simulink model "TP2_R3FMO_ctrl_2016"  (R2017b)
settings: Solver=ode23s  StartTime=0.0  StopTime=.15  RelTol=1e-3  EnableMultiTasking=on
values from neighbouring files (symbols this model uses):
  anchoPulso = 5    [TP2_R3FMO_ctrl_2016.m]    (also in TP2_R3FMO_ctrl_2016_p_2.m = 40; TP2_R3FMO_ctrl_2016_p_3.m = 40)
  t1 = fase1+theta    (= 0.00666666666667)    [TP2_R3FMO_ctrl_2016.m]    (also in TP2_R3FMO_ctrl_2016_p_2.m = 0.005; TP2_R3FMO_ctrl_2016_p_3.m = 0.005)
  t2 = fase2+theta    (= 0.0133333333333)    [TP2_R3FMO_ctrl_2016.m]    (also in TP2_R3FMO_ctrl_2016_p_2.m = 0.0116666666667; TP2_R3FMO_ctrl_2016_p_3.m = 0.0116666666667)
  t3 = fase3+theta    (= 0.02)    [TP2_R3FMO_ctrl_2016.m]    (also in TP2_R3FMO_ctrl_2016_p_2.m = 0.0183333333333; TP2_R3FMO_ctrl_2016_p_3.m = 0.0183333333333)
  tCorto = 0.075    [TP2_R3FMO_ctrl_2016.m]    (also in TP2_R3FMO_ctrl_2016_p_2.m = 0.028; TP2_R3FMO_ctrl_2016_p_3.m = 0.028)
libraries: powerlib x11, powerlib_meascontrol x2
settings Model: Creator=Moni  LastModifiedBy=Sebastián
settings DataIOCC: SaveFormat=Array  SaveState=on
settings OptimizationCC: LifeSpan=inf
settings DebuggingCC: SolverPrmCheckMsg=warning  SFUnexpectedBacktrackingDiag=warning  SFNoUnconditionalDefaultTransitionDiag=warning  SFExecutionAtInitializationDiag=none
settings HardwareCC: ProdBitPerPointer=32  ProdBitPerSizeT=32  ProdBitPerPtrDiffT=32  ProdLargestAtomicFloat=None  ProdIntDivRoundTo=Undefined  ProdEndianess=Unspecified  ProdWordSize=32  ProdHWDeviceType=32-bit Generic
settings ModelReferenceCC: PropagateSignalLabelsOutOfModel=off
settings CodeAppCC: StateflowObjectComments=on
settings GRTTargetCC: TargetLangStandard=C89/C90 (ANSI)  GeneratePreprocessorConditionals=Disable all
settings ConfigComp: CovMetricSettings=dw  CovHtmlReporting=on  CovSaveCumulativeToWorkspaceVar=on  CovSaveSingleToWorkspaceVar=on  CovExternalEMLEnable=off  CovSFcnEnable=off
settings SimscapeCC: SimscapeNormalizeSystem=off

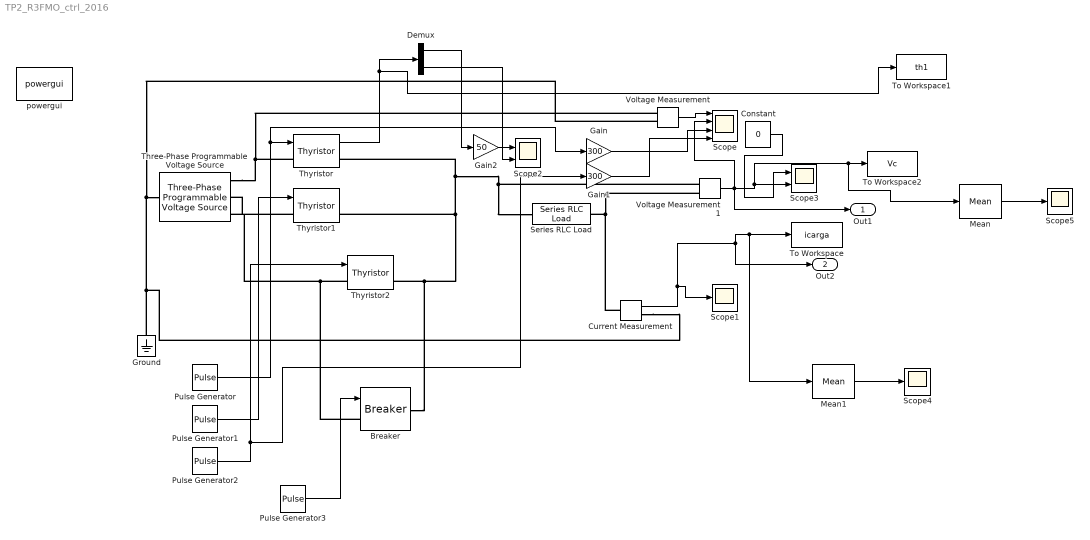
== system TP2_R3FMO_ctrl_2016 ==
  Breaker : powerlib/Elements/Breaker  InitialState=0  SwitchingTimes="[1/60  5/60]"  External=on  BreakerResistance=0.01  SnubberResistance=1e6  SnubberCapacitance=inf  Measurements=None  MoreParameters=on  NoBreakLoop=off
      settings: SourceProductName=Simscape Power Systems
  Constant : Constant  Value=0
  Current Measurement : powerlib/Measurements/Current Measurement  PhasorSimulation=off  OutputType=Complex  PSBequivalent=0
  Demux : Demux  Outputs=2
  Gain : Gain  Gain=300
  Gain1 : Gain  Gain=300
  Gain2 : Gain  Gain=50
  Ground : powerlib/Elements/Ground  LConnTagsString=a
  Mean : powerlib_meascontrol/Measurements/Mean  Freq=50  Vinit=0  Ts=0
  Mean1 : powerlib_meascontrol/Measurements/Mean  Freq=50  Vinit=0  Ts=0
  Pulse Generator : DiscretePulseGenerator  PulseType=Time based  Period=.02  PulseWidth=anchoPulso  PhaseDelay=t1
  Pulse Generator1 : DiscretePulseGenerator  PulseType=Time based  Period=.02  PulseWidth=anchoPulso  PhaseDelay=t2
  Pulse Generator2 : DiscretePulseGenerator  PulseType=Time based  Period=.02  PulseWidth=anchoPulso  PhaseDelay=t3
  Pulse Generator3 : DiscretePulseGenerator  PulseType=Time based  Period=10  PulseWidth=99  PhaseDelay=tCorto
  Scope : Scope  NumInputPorts=4
  Scope1 : Scope
  Scope2 : Scope  NumInputPorts=2
  Scope3 : Scope  NumInputPorts=2
  Scope4 : Scope
  Scope5 : Scope
  Series RLC Load : powerlib/Elements/Series RLC Load  LConnTagsString=a  RConnTagsString=__new0  NominalVoltage=220  NominalFrequency=50  ActivePower=100  InductivePower=Q  CapacitivePower=0  Setx0=off  InitialVoltage=0  SetiL0=off  InitialCurrent=0  Measurements=None  LoadType=constant Z
  Three-Phase Programmable Voltage Source : powerlib/Electrical Sources/Three-Phase Programmable Voltage Source  PositiveSequence="[380  0 50]"  VariationEntity=None  VariationType=Table of time-amplitude pairs  VariationTypeAlt=Step  VariationStep=0.5  VariationRate=10  VariationMagnitude=0.3  VariationFrequency=2  VariationTiming=[1 2]  VariationPhaseA=off  Amplitudes=[1 0.8 1.2 1.0]  TimeValues=[0 0.1 0.15 0.2]  HarmonicGeneration=off  HarmonicA=[3 0.2 -25 0]  HarmonicB=[2 0.15 35 2]  Timing="[0.05  3]"  BusType=swing  Pref=0  Qref=0  Qmin=-inf  Qmax=inf
  Thyristor : powerlib/Power Electronics/Thyristor  Ron=0.001  Lon=0  Vf=0.8  IC=0  Rs=400  Cs=C  Measurements=on
  Thyristor1 : powerlib/Power Electronics/Thyristor  Ron=0.001  Lon=0  Vf=0.8  IC=0  Rs=400  Cs=C  Measurements=on
  Thyristor2 : powerlib/Power Electronics/Thyristor  Ron=0.001  Lon=0  Vf=0.8  IC=0  Rs=400  Cs=C  Measurements=on
  To Workspace : ToWorkspace  VariableName=icarga  SampleTime=-1
  To Workspace1 : ToWorkspace  VariableName=th1  SampleTime=-1
  To Workspace2 : ToWorkspace  VariableName=Vc  SampleTime=-1
  Voltage Measurement : powerlib/Measurements/Voltage Measurement  PhasorSimulation=off  OutputType=Complex  PSBequivalent=0
  Voltage Measurement1 : powerlib/Measurements/Voltage Measurement  PhasorSimulation=off  OutputType=Complex  PSBequivalent=0
  powergui : powerlib/powergui  Priority=1  SimulationMode=Continuous  SampleTime=50e-6  frequency=60  Iterations=50  frequencyindice=50  Pbase=100e6  ErrMax=1e-4  UnitsV=kV  UnitsW=MW  buscounter=0  FunctionMessages=off  echomessages=off  EnableUseOfTLC=off  CurrentSourceSwitches=on  DisableSnubberDevices=off  DisableRonSwitches=off  DisableVfSwitches=off  DisplayEquations=off  SolverType=Tustin  Interpol=off  ExternalGateDelay=off  methode=off  Ts=0  x0status=blocks  SPID=off  SwTol=0  HookPort=off  RestoreLinks=warning  ResistiveCurrentMeasurement=off  Frange=[0:2:500]  Ylog=off  Xlog=on  ShowGrid=off  save=off  variable=ZData  structure=Vc  ZoomFFT=off  StartTime=0.3  cycles=3  DisplayStyle=1  fundamental=50  FreqAxis=off  MaxFrequency=500  frequencyindicesteady=1  RmsSteady=1  display=off
  Out1 : Outport
  Out2 : Outport  Port=2
  wires:
  Voltage Measurement/1 -> Scope/1
  Current Measurement/1 -> Scope1/1, Out2/1, Mean1/1, To Workspace/1
  Voltage Measurement1/1 -> Scope/2, Out1/1, Scope3/2, Mean/1, To Workspace2/1
  Mean1/1 -> Scope4/1
  Mean/1 -> Scope5/1
  Pulse Generator/1 -> Gain/1, Thyristor/1
  Gain/1 -> Scope/3
  Pulse Generator1/1 -> Thyristor1/1
  Gain1/1 -> Scope/4
  Pulse Generator2/1 -> Gain1/1, Thyristor2/1
  Constant/1 -> Scope3/1
  Demux/2 -> Scope2/2
  Demux/1 -> Gain2/1
  Gain2/1 -> Scope2/1
  Pulse Generator3/1 -> Breaker/1
  Thyristor/1 -> To Workspace1/1, Demux/1
  connections:
  Three-Phase Programmable Voltage Source/RConn1 -- Thyristor/LConn1 -- Voltage Measurement/LConn1
  Thyristor1/LConn1 -- Three-Phase Programmable Voltage Source/RConn2
  Thyristor2/LConn1 -- Breaker/LConn1 -- Three-Phase Programmable Voltage Source/RConn3
  Ground/LConn1 -- Current Measurement/RConn1 -- Voltage Measurement/LConn2 -- Three-Phase Programmable Voltage Source/LConn1
  Breaker/RConn1 -- Thyristor2/RConn1 -- Thyristor1/RConn1 -- Thyristor/RConn1 -- Voltage Measurement1/LConn1 -- Series RLC Load/LConn1
  Current Measurement/LConn1 -- Voltage Measurement1/LConn2 -- Series RLC Load/RConn1
